simulink library "cmmi_lib"  (R2024a)
settings: Solver=VariableStepAuto  StartTime=0.0  StopTime=10.0  RelTol=1e-3
undefined symbols (not defined in the file): alloc_B, Keff, ss_x, ss_yaw, t200, t200_force_n, t200_pwm_n, Ts
libraries: ros2lib x12, MarineRoboticsLib x2, robotcorelib x1
settings Model: Creator=luka  LastModifiedBy=luka

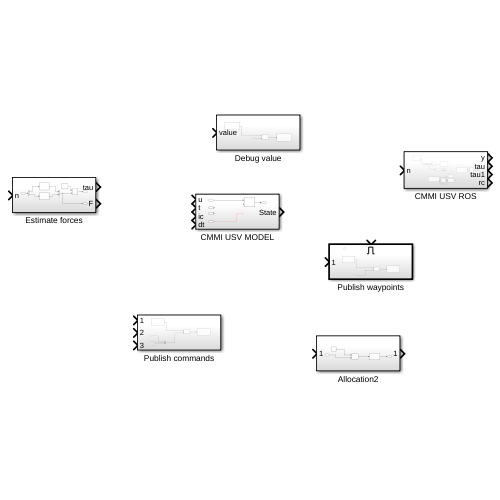
[thumbnail: Simulink's stored preview of the top-level diagram]
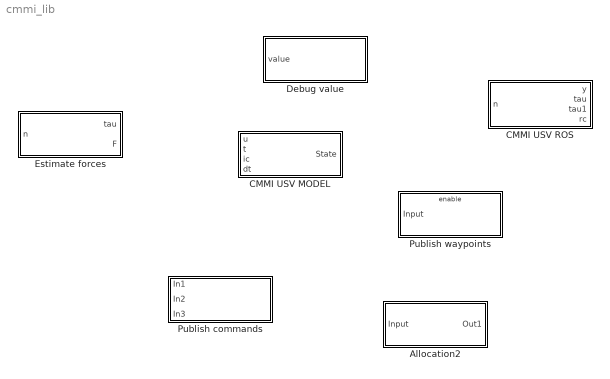
== system cmmi_lib ==
  Allocation2 : Subsystem
  CMMI USV MODEL : Subsystem
  CMMI USV ROS : Subsystem
  Debug value : Subsystem
  Estimate forces : Subsystem
  Publish commands : Subsystem
  Publish waypoints : Subsystem  TreatAsAtomicUnit=on

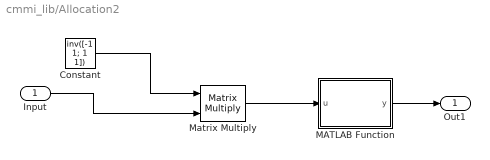
== system cmmi_lib/Allocation2 ==
  Input : Inport
  Constant : Constant  Value=inv([-1 1; 1 1])
  MATLAB Function : MATLAB Function  TreatAsAtomicUnit=on
  Matrix Multiply : Product  Multiplication=Matrix(*)
  Out1 : Outport
  wires:
  MATLAB Function/1(y) -> Out1/1
  Matrix Multiply/1 -> MATLAB Function/1(u)
  Input/1 -> Matrix Multiply/2
  Constant/1 -> Matrix Multiply/1

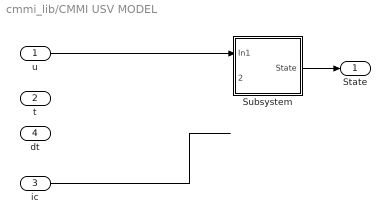
== system cmmi_lib/CMMI USV MODEL ==
  u : Inport
  t : Inport  Port=2
  ic : Inport  Port=3
  dt : Inport  Port=4
  Subsystem : Subsystem
  State : Outport
  wires:
  u/1 -> Subsystem/1(In1)
  Subsystem/1(State) -> State/1
  ic/1 -> ?

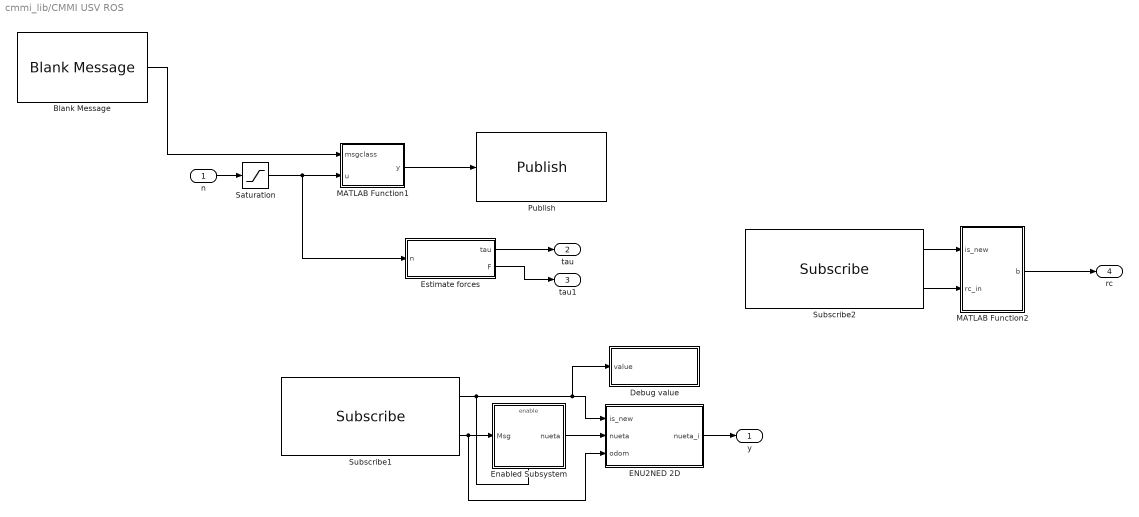
== system cmmi_lib/CMMI USV ROS ==
  n : Inport
  Blank Message : ros2lib/Blank Message  messageClass=Message  entityType=std_msgs/Float32MultiArray  messageType=std_msgs/Float32MultiArray  SampleTime=Ts
  Debug value : Subsystem  AncestorBlock=cmmi_lib/Debug value
  ENU2NED 2D : MATLAB Function  TreatAsAtomicUnit=on
  Enabled Subsystem : Subsystem  TreatAsAtomicUnit=on
  Estimate forces : Subsystem  AncestorBlock=cmmi_lib/Estimate forces
  MATLAB Function1 : MATLAB Function  TreatAsAtomicUnit=on
  MATLAB Function2 : MATLAB Function  TreatAsAtomicUnit=on  SystemSampleTime=Ts
  Publish : ros2lib/Publish  topicSource=Specify your own  topic=/pwm_in  messageType=std_msgs/Float32MultiArray  QOSHistory=Keep last  QOSDepth=1  QOSReliability=Reliable  QOSDurability=Volatile  QOSDeadline=Inf  QOSLifespan=Inf  QOSLiveliness=Automatic  QOSLeaseDuration=Inf  QOSAvoidROSNamespaceConventions=off
  Saturation : Saturate  UpperLimit=1  LowerLimit=-1
  Subscribe1 : ros2lib/Subscribe  topicSource=Specify your own  topic=/mavros/local_position/odom  messageType=nav_msgs/Odometry  sampleTime=0.05  QOSHistory=Keep last  QOSDepth=1  QOSReliability=Best effort  QOSDurability=Volatile  QOSDeadline=Inf  QOSLifespan=Inf  QOSLiveliness=Automatic  QOSLeaseDuration=Inf  QOSAvoidROSNamespaceConventions=off
  Subscribe2 : ros2lib/Subscribe  topicSource=Specify your own  topic=/rc_btns  messageType=std_msgs/Int8MultiArray  sampleTime=Ts  QOSHistory=Keep all  QOSDepth=1  QOSReliability=Best effort  QOSDurability=Volatile  QOSDeadline=Inf  QOSLifespan=Inf  QOSLiveliness=Automatic  QOSLeaseDuration=Inf  QOSAvoidROSNamespaceConventions=off
  y : Outport
  tau : Outport  Port=2
  tau1 : Outport  Port=3
  rc : Outport  Port=4
  wires:
  Saturation/1 -> MATLAB Function1/2(u), Estimate forces/1(n)
  ENU2NED 2D/1(nueta_i) -> y/1
  Enabled Subsystem/1(nueta) -> ENU2NED 2D/2(nueta)
  Subscribe1/1 -> Enabled Subsystem/Enable, ENU2NED 2D/1(is_new), Debug value/1(value)
  Subscribe1/2 -> Enabled Subsystem/1(Msg), ENU2NED 2D/3(odom)
  MATLAB Function2/1(b) -> rc/1
  Subscribe2/2 -> MATLAB Function2/2(rc_in)
  Subscribe2/1 -> MATLAB Function2/1(is_new)
  n/1 -> Saturation/1
  Blank Message/1 -> MATLAB Function1/1(msgclass)
  MATLAB Function1/1(y) -> Publish/1
  Estimate forces/1(tau) -> tau/1
  Estimate forces/2(F) -> tau1/1

== system cmmi_lib/Debug value ==
  value : Inport
  Blank Message : ros2lib/Blank Message  messageClass=Message  entityType=std_msgs/Float32MultiArray  messageType=std_msgs/Float32MultiArray  SampleTime=Ts
  MATLAB Function1 : MATLAB Function  TreatAsAtomicUnit=on
  Publish : ros2lib/Publish  topicSource=Specify your own  topic=debug  messageType=std_msgs/Float32MultiArray  QOSHistory=Keep last  QOSDepth=1  QOSReliability=Reliable  QOSDurability=Volatile  QOSDeadline=Inf  QOSLifespan=Inf  QOSLiveliness=Automatic  QOSLeaseDuration=Inf  QOSAvoidROSNamespaceConventions=off
  wires:
  value/1 -> MATLAB Function1/2(u)
  Blank Message/1 -> MATLAB Function1/1(msgclass)
  MATLAB Function1/1(y) -> Publish/1

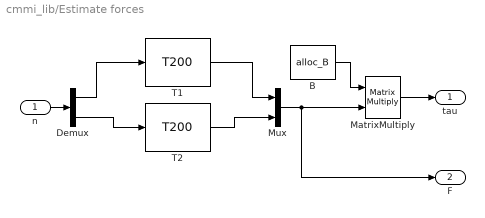
== system cmmi_lib/Estimate forces ==
  n : Inport
  B : Constant  Value=alloc_B
  Demux : Demux  Outputs=2
  MatrixMultiply : Product  Multiplication=Matrix(*)
  Mux : Mux  Inputs=2
  T1 : MarineRoboticsLib/T200  Keff=Keff(1)  Tm=Tm
  T2 : MarineRoboticsLib/T200  Keff=Keff(2)  Tm=Tm
  tau : Outport
  F : Outport  Port=2
  wires:
  MatrixMultiply/1 -> tau/1
  Demux/2 -> T2/1
  n/1 -> Demux/1
  Demux/1 -> T1/1
  Mux/1 -> MatrixMultiply/2, F/1
  T2/1 -> Mux/2
  B/1 -> MatrixMultiply/1
  T1/1 -> Mux/1

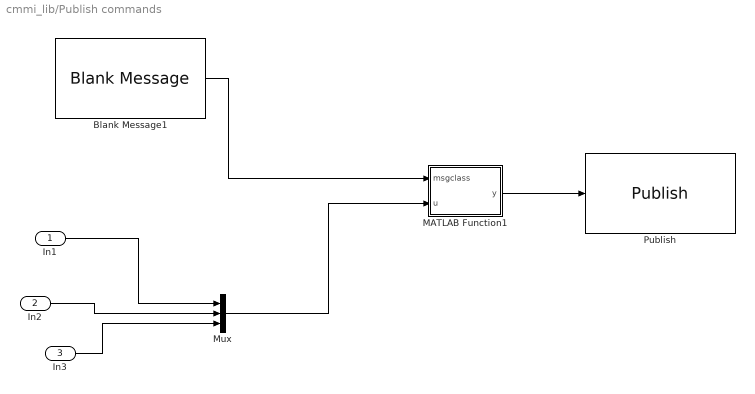
== system cmmi_lib/Publish commands ==
  In1 : Inport
  In2 : Inport  Port=2
  In3 : Inport  Port=3
  Blank Message1 : ros2lib/Blank Message  messageClass=Message  entityType=std_msgs/Float32MultiArray  messageType=std_msgs/Float32MultiArray  SampleTime=Ts
  MATLAB Function1 : MATLAB Function  TreatAsAtomicUnit=on
  Mux : Mux  Inputs=3
  Publish : ros2lib/Publish  topicSource=Specify your own  topic=/commands  messageType=std_msgs/Float32MultiArray  QOSHistory=Keep last  QOSDepth=1  QOSReliability=Reliable  QOSDurability=Volatile  QOSDeadline=Inf  QOSLifespan=Inf  QOSLiveliness=Automatic  QOSLeaseDuration=Inf  QOSAvoidROSNamespaceConventions=off
  wires:
  Blank Message1/1 -> MATLAB Function1/1(msgclass)
  MATLAB Function1/1(y) -> Publish/1
  Mux/1 -> MATLAB Function1/2(u)
  In1/1 -> Mux/1
  In2/1 -> Mux/2
  In3/1 -> Mux/3

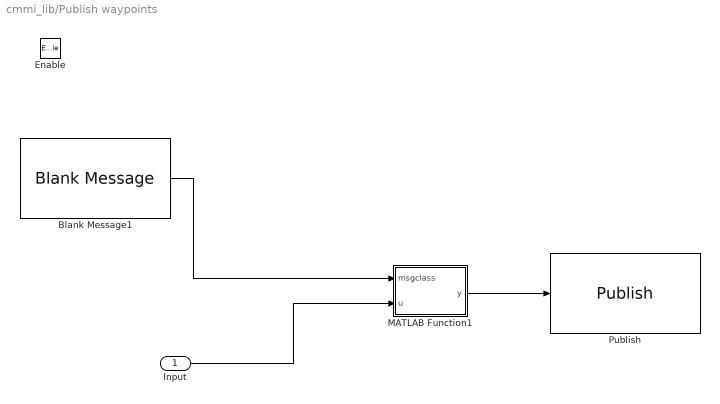
== system cmmi_lib/Publish waypoints ==
  Input : Inport
  Enable : EnablePort
  Blank Message1 : ros2lib/Blank Message  messageClass=Message  entityType=nav_msgs/Path  messageType=nav_msgs/Path  SampleTime=1
  MATLAB Function1 : MATLAB Function  TreatAsAtomicUnit=on
  Publish : ros2lib/Publish  topicSource=Specify your own  topic=/waypoints  messageType=nav_msgs/Path  QOSHistory=Keep last  QOSDepth=1  QOSReliability=Reliable  QOSDurability=Volatile  QOSDeadline=Inf  QOSLifespan=Inf  QOSLiveliness=Automatic  QOSLeaseDuration=Inf  QOSAvoidROSNamespaceConventions=off
  wires:
  Blank Message1/1 -> MATLAB Function1/1(msgclass)
  Input/1 -> MATLAB Function1/2(u)
  MATLAB Function1/1(y) -> Publish/1

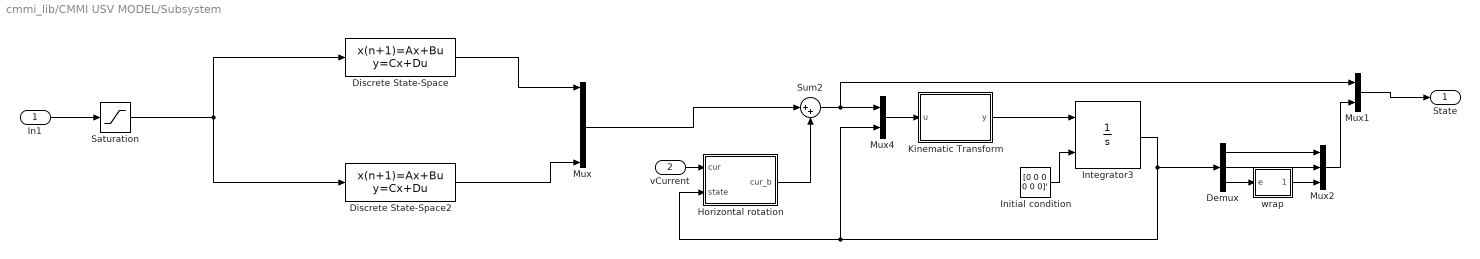
== system cmmi_lib/CMMI USV MODEL/Subsystem ==
  In1 : Inport
  vCurrent : Inport  Port=2
  Demux : Demux  Outputs=3
  Discrete State-Space : DiscreteStateSpace  A=ss_x.A  B=ss_x.B  C=ss_x.C  D=ss_x.D  SampleTime=ss_x.Ts
  Discrete State-Space2 : DiscreteStateSpace  A=ss_yaw.A  B=ss_yaw.B  C=ss_yaw.C  D=ss_yaw.D  SampleTime=ss_yaw.Ts
  Horizontal rotation : MATLAB Function  TreatAsAtomicUnit=on
  Initial condition : Constant  Value=[0 0 0 0 0 0]'
  Integrator3 : Integrator  InitialConditionSource=external
  Kinematic Transform : MATLAB Function  TreatAsAtomicUnit=on
  Mux : Mux  Inputs=6
  Mux1 : Mux  Inputs=2
  Mux2 : Mux  Inputs=3
  Mux4 : Mux  Inputs=2
  Saturation : Saturate  UpperLimit=1  LowerLimit=-1
  Sum2 : Sum  Inputs=|++
  wrap : MATLAB Function  TreatAsAtomicUnit=on
  State : Outport
  wires:
  In1/1 -> Saturation/1
  Discrete State-Space2/1 -> Mux/6
  Kinematic Transform/1(y) -> Integrator3/1
  Initial condition/1 -> Integrator3/2
  Sum2/1 -> Mux1/1, Mux4/1
  vCurrent/1 -> Horizontal rotation/1(cur)
  Mux4/1 -> Kinematic Transform/1(u)
  Integrator3/1 -> Demux/1, Horizontal rotation/2(state), Mux4/2
  Mux/1 -> Sum2/1
  Horizontal rotation/1(cur_b) -> Sum2/2
  Mux1/1 -> State/1
  Discrete State-Space/1 -> Mux/1
  Demux/3 -> wrap/1(e)
  wrap/1(ew) -> Mux2/3
  Demux/1 -> Mux2/1
  Demux/2 -> Mux2/2
  Mux2/1 -> Mux1/2
  Saturation/1 -> Discrete State-Space2/1, Discrete State-Space/1

== system cmmi_lib/CMMI USV ROS/Debug value ==
  value : Inport
  Blank Message : ros2lib/Blank Message  messageClass=Message  entityType=std_msgs/Float32MultiArray  messageType=std_msgs/Float32MultiArray  SampleTime=Ts
  MATLAB Function1 : MATLAB Function  TreatAsAtomicUnit=on
  Publish : ros2lib/Publish  topicSource=Specify your own  topic=debug_isnew  messageType=std_msgs/Float32MultiArray  QOSHistory=Keep last  QOSDepth=1  QOSReliability=Reliable  QOSDurability=Volatile  QOSDeadline=Inf  QOSLifespan=Inf  QOSLiveliness=Automatic  QOSLeaseDuration=Inf  QOSAvoidROSNamespaceConventions=off
  wires:
  MATLAB Function1/1(y) -> Publish/1
  Blank Message/1 -> MATLAB Function1/1(msgclass)
  value/1 -> MATLAB Function1/2(u)

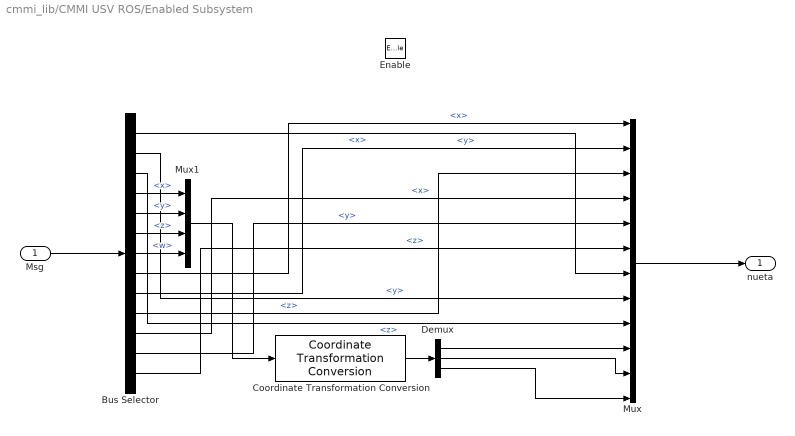
== system cmmi_lib/CMMI USV ROS/Enabled Subsystem ==
  Msg : Inport
  Enable : EnablePort
  Bus Selector : BusSelector  OutputSignals=pose.pose.position.x,pose.pose.position.y,pose.pose.position.z,pose.pose.orientation.x,pose.pose.orientation.y,pose.pose.orientation.z,pose.pose.orientation.w,twist.twist.linear.x,twist.twist.linear.y,twist.twist.linear.z,twist.twist.angular.x,twist.twist.angular.y,twist.twist.angular.z
  Coordinate Transformation Conversion : robotcorelib/Coordinate Transformation Conversion  InputRepresentation=Quaternion  InputEulerSequence=ZYX  ShowTrVecInputPort=on  OutputRepresentation=Euler Angles  OutputEulerSequence=ZYX  ShowTrVecOutputPort=on  SimulateUsing=Code generation
      settings: LibrarySourceBlock=roslib/Utilities/Coordinate Transformation Conversion
  Demux : Demux  Outputs=3
  Mux : Mux  Inputs=12
  Mux1 : Mux
  nueta : Outport
  wires:
  Bus Selector/12 -> Mux/5  "<y>"
  Bus Selector/11 -> Mux/4  "<x>"
  Bus Selector/10 -> Mux/3  "<z>"
  Demux/1 -> Mux/10
  Demux/2 -> Mux/11
  Bus Selector/3 -> Mux/9  "<z>"
  Msg/1 -> Bus Selector/1
  Bus Selector/4 -> Mux1/1  "<x>"
  Bus Selector/5 -> Mux1/2  "<y>"
  Bus Selector/6 -> Mux1/3  "<z>"
  Bus Selector/7 -> Mux1/4  "<w>"
  Mux1/1 -> Coordinate Transformation Conversion/1
  Bus Selector/2 -> Mux/8  "<y>"
  Bus Selector/1 -> Mux/7  "<x>"
  Coordinate Transformation Conversion/1 -> Demux/1
  Bus Selector/8 -> Mux/1  "<x>"
  Bus Selector/9 -> Mux/2  "<y>"
  Bus Selector/13 -> Mux/6  "<z>"
  Mux/1 -> nueta/1
  Demux/3 -> Mux/12

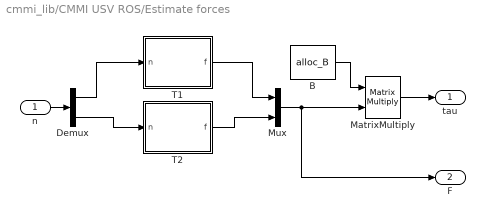
== system cmmi_lib/CMMI USV ROS/Estimate forces ==
  n : Inport
  B : Constant  Value=alloc_B
  Demux : Demux  Outputs=2
  MatrixMultiply : Product  Multiplication=Matrix(*)
  Mux : Mux  Inputs=2
  T1 : Subsystem  mask(T200){Keff=t200(1).Keff, Tm=t200(1).Tm}
      mask prompts: Keff "Efficiency"; Tm "ESC time constant (Tm)"
      mask help: This simulink block simulates a Blue Robotics T200 thruster on 14V controlled input. The efficiancy parameter given from [0,1] additionally decreases the force output of the thruster. The ESC reaction time is the time constant of the PT1 element included in the model. Put the time constant to zero to have instantaneous response.
      mask Display: image('$imagefile'); % Use "Edit Image" on toolstrip to change.
  T2 : Subsystem  mask(T200){Keff=t200(2).Keff, Tm=t200(2).Tm}
      mask prompts: Keff "Efficiency"; Tm "ESC time constant (Tm)"
      mask help: This simulink block simulates a Blue Robotics T200 thruster on 14V controlled input. The efficiancy parameter given from [0,1] additionally decreases the force output of the thruster. The ESC reaction time is the time constant of the PT1 element included in the model. Put the time constant to zero to have instantaneous response.
      mask Display: image('$imagefile'); % Use "Edit Image" on toolstrip to change.
  tau : Outport
  F : Outport  Port=2
  wires:
  T1/1(f) -> Mux/1
  B/1 -> MatrixMultiply/1
  T2/1(f) -> Mux/2
  Mux/1 -> F/1, MatrixMultiply/2
  Demux/1 -> T1/1(n)
  n/1 -> Demux/1
  Demux/2 -> T2/1(n)
  MatrixMultiply/1 -> tau/1

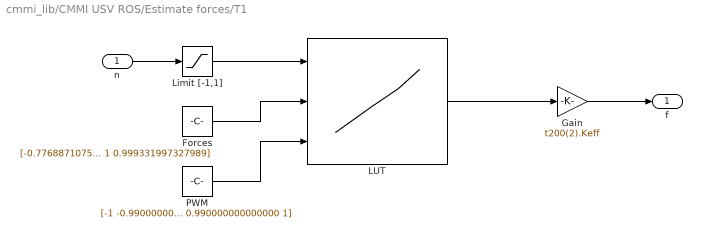
== system cmmi_lib/CMMI USV ROS/Estimate forces/T1 ==
  n : Inport
  Forces : Constant  Value=|
      | [-0.776887107548430
      | -0.772545090180361
      | -0.771543086172345
      | -0.762525050100200
      | -0.751503006012024
      | -0.741482965931864
      | -0.727454909819639
      | -0.717434869739479
      | -0.704408817635270
      | -0.693386773547094
      | -0.684368737474950
      | -0.675350701402806
      | -0.663326653306613
      | -0.649298597194389
      | -0.637274549098196
      | -0.629258517034068
      | -0.614228456913828
      | -0.610220440881764
      | -0.594188376753507
      | -0.584168336673347
      | -0.573146292585170
      | -0.558116232464930
      | -0.550100200400802
      | -0.542084168336673
      | -0.532064128256513
      | -0.519038076152305
      | -0.516032064128256
      | -0.498997995991984
      | -0.486973947895792
      | -0.480961923847695
      | -0.467935871743487
      | -0.453907815631262
      | -0.447895791583166
      | -0.438877755511022
      | -0.421843687374750
      | -0.417835671342685
      | -0.401803607214429
      | -0.389779559118237
      | -0.379759519038076
      | -0.371743486973948
      | -0.360721442885772
      | -0.348697394789579
      | -0.345691382765531
      | -0.335671342685371
      | -0.326653306613226
      | -0.318637274549098
      | -0.309619238476954
      | -0.302605210420842
      | -0.292585170340681
      | -0.283567134268537
      | -0.273547094188377
      | -0.263527054108217
      | -0.257515030060120
      | -0.248496993987976
      | -0.240480961923848
      | -0.232464929859719
      | -0.224448897795591
      | -0.217434869739479
      | -0.210420841683367
      | -0.202404809619238
      | -0.195390781563126
      | -0.187374749498998
      | -0.178356713426854
      | -0.169338677354709
      | -0.163326653306613
      | -0.155310621242485
      | -0.150300601202405
      | -0.143286573146293
      | -0.137274549098196
      | -0.129258517034068
      | -0.121242484969940
      | -0.114228456913828
      | -0.108216432865731
      | -0.102204408817635
      | -0.0941883767535070
      | -0.0881763527054108
      | -0.0821643286573146
      | -0.0771543086172345
      | -0.0701402805611222
      | -0.0631262525050100
      | -0.0571142284569138
      | -0.0521042084168337
      | -0.0460921843687375
      | -0.0410821643286573
      | -0.0360721442885772
      | -0.0320641282565130
      | -0.0270541082164329
      | -0.0220440881763527
      | -0.0180360721442886
      | -0.0150300601202405
      | -0.0100200400801603
      | -0.00701402805611223
      | 0
      | 0
      | 0
      | 0
      | 0
      | 0
      | 0
      | 0
      | 0
      | 0
      | 0
      | 0
      | 0
      | 0
      | 0
      | 0
      | 0
      | 0.0100200400801603
      | 0.0140280561122245
      | 0.0180360721442886
      | 0.0220440881763527
      | 0.0270541082164329
      | 0.0320641282565130
      | 0.0390781563126253
      | 0.0440881763527054
      | 0.0501002004008016
      | 0.0581162324649299
      | 0.0641282565130261
      | 0.0721442885771543
      | 0.0801603206412826
      | 0.0871743486973948
      | 0.0941883767535070
      | 0.102204408817635
      | 0.110220440881764
      | 0.117234468937876
      | 0.127254509018036
      | 0.137274549098196
      | 0.142284569138277
      | 0.152304609218437
      | 0.160320641282565
      | 0.169338677354709
      | 0.182364729458918
      | 0.187374749498998
      | 0.196392785571142
      | 0.203406813627254
      | 0.213426853707415
      | 0.220440881763527
      | 0.232464929859719
      | 0.241482965931864
      | 0.252505010020040
      | 0.265531062124249
      | 0.272545090180361
      | 0.282565130260521
      | 0.292585170340681
      | 0.301603206412826
      | 0.310621242484970
      | 0.322645290581162
      | 0.333667334669339
      | 0.342685370741483
      | 0.354709418837675
      | 0.364729458917836
      | 0.377755511022044
      | 0.388777555110220
      | 0.400801603206413
      | 0.408817635270541
      | 0.421843687374750
      | 0.433867735470942
      | 0.442885771543086
      | 0.460921843687375
      | 0.467935871743487
      | 0.476953907815631
      | 0.495991983967936
      | 0.501002004008016
      | 0.517034068136273
      | 0.536072144288577
      | 0.553106212424850
      | 0.566132264529058
      | 0.582164328657315
      | 0.587174348697395
      | 0.609218436873748
      | 0.614228456913828
      | 0.636272545090180
      | 0.648296593186373
      | 0.661322645290581
      | 0.673346693386774
      | 0.691382765531062
      | 0.704408817635271
      | 0.714428857715431
      | 0.734468937875751
      | 0.742484969939880
      | 0.755511022044088
      | 0.771543086172345
      | 0.787575150300601
      | 0.800601202404810
      | 0.814629258517034
      | 0.832665330661323
      | 0.847695390781563
      | 0.866733466933868
      | 0.879759519038076
      | 0.889779559118237
      | 0.907815631262525
      | 0.917835671342685
      | 0.930861723446894
      | 0.950901803607214
      | 0.967935871743487
      | 0.976953907815631
      | 0.995991983967936
      | 1
      | 0.999331997327989]
  Gain : Gain  Gain=t200(2).Keff
  LUT : Lookup_n-D  NumberOfTableDimensions=1  BreakpointsForDimension1Source=Input port  BreakpointsForDimension1=t200_pwm_n  TableSource=Input port  Table=t200_force_n  InternalRulePriority=Speed  RndMeth=Simplest
      settings: InputPortMap=u0,p221,p5
  Limit [-1,1] : Saturate  UpperLimit=1  LowerLimit=-1
  PWM : Constant  Value=|
      | [-1
      | -0.990000000000000
      | -0.980000000000000
      | -0.970000000000000
      | -0.960000000000000
      | -0.950000000000000
      | -0.940000000000000
      | -0.930000000000000
      | -0.920000000000000
      | -0.910000000000000
      | -0.900000000000000
      | -0.890000000000000
      | -0.880000000000000
      | -0.870000000000000
      | -0.860000000000000
      | -0.850000000000000
      | -0.840000000000000
      | -0.830000000000000
      | -0.820000000000000
      | -0.810000000000000
      | -0.800000000000000
      | -0.790000000000000
      | -0.780000000000000
      | -0.770000000000000
      | -0.760000000000000
      | -0.750000000000000
      | -0.740000000000000
      | -0.730000000000000
      | -0.720000000000000
      | -0.710000000000000
      | -0.700000000000000
      | -0.690000000000000
      | -0.680000000000000
      | -0.670000000000000
      | -0.660000000000000
      | -0.650000000000000
      | -0.640000000000000
      | -0.630000000000000
      | -0.620000000000000
      | -0.610000000000000
      | -0.600000000000000
      | -0.590000000000000
      | -0.580000000000000
      | -0.570000000000000
      | -0.560000000000000
      | -0.550000000000000
      | -0.540000000000000
      | -0.530000000000000
      | -0.520000000000000
      | -0.510000000000000
      | -0.500000000000000
      | -0.490000000000000
      | -0.480000000000000
      | -0.470000000000000
      | -0.460000000000000
      | -0.450000000000000
      | -0.440000000000000
      | -0.430000000000000
      | -0.420000000000000
      | -0.410000000000000
      | -0.400000000000000
      | -0.390000000000000
      | -0.380000000000000
      | -0.370000000000000
      | -0.360000000000000
      | -0.350000000000000
      | -0.340000000000000
      | -0.330000000000000
      | -0.320000000000000
      | -0.310000000000000
      | -0.300000000000000
      | -0.290000000000000
      | -0.280000000000000
      | -0.270000000000000
      | -0.260000000000000
      | -0.250000000000000
      | -0.240000000000000
      | -0.230000000000000
      | -0.220000000000000
      | -0.210000000000000
      | -0.200000000000000
      | -0.190000000000000
      | -0.180000000000000
      | -0.170000000000000
      | -0.160000000000000
      | -0.150000000000000
      | -0.140000000000000
      | -0.130000000000000
      | -0.120000000000000
      | -0.110000000000000
      | -0.100000000000000
      | -0.0900000000000000
      | -0.0800000000000000
      | -0.0700000000000000
      | -0.0600000000000000
      | -0.0500000000000000
      | -0.0400000000000000
      | -0.0300000000000000
      | -0.0200000000000000
      | -0.0100000000000000
      | 0
      | 0.0100000000000000
      | 0.0200000000000000
      | 0.0300000000000000
      | 0.0400000000000000
      | 0.0500000000000000
      | 0.0600000000000000
      | 0.0700000000000000
      | 0.0800000000000000
      | 0.0900000000000000
      | 0.100000000000000
      | 0.110000000000000
      | 0.120000000000000
      | 0.130000000000000
      | 0.140000000000000
      | 0.150000000000000
      | 0.160000000000000
      | 0.170000000000000
      | 0.180000000000000
      | 0.190000000000000
      | 0.200000000000000
      | 0.210000000000000
      | 0.220000000000000
      | 0.230000000000000
      | 0.240000000000000
      | 0.250000000000000
      | 0.260000000000000
      | 0.270000000000000
      | 0.280000000000000
      | 0.290000000000000
      | 0.300000000000000
      | 0.310000000000000
      | 0.320000000000000
      | 0.330000000000000
      | 0.340000000000000
      | 0.350000000000000
      | 0.360000000000000
      | 0.370000000000000
      | 0.380000000000000
      | 0.390000000000000
      | 0.400000000000000
      | 0.410000000000000
      | 0.420000000000000
      | 0.430000000000000
      | 0.440000000000000
      | 0.450000000000000
      | 0.460000000000000
      | 0.470000000000000
      | 0.480000000000000
      | 0.490000000000000
      | 0.500000000000000
      | 0.510000000000000
      | 0.520000000000000
      | 0.530000000000000
      | 0.540000000000000
      | 0.550000000000000
      | 0.560000000000000
      | 0.570000000000000
      | 0.580000000000000
      | 0.590000000000000
      | 0.600000000000000
      | 0.610000000000000
      | 0.620000000000000
      | 0.630000000000000
      | 0.640000000000000
      | 0.650000000000000
      | 0.660000000000000
      | 0.670000000000000
      | 0.680000000000000
      | 0.690000000000000
      | 0.700000000000000
      | 0.710000000000000
      | 0.720000000000000
      | 0.730000000000000
      | 0.740000000000000
      | 0.750000000000000
      | 0.760000000000000
      | 0.770000000000000
      | 0.780000000000000
      | 0.790000000000000
      | 0.800000000000000
      | 0.810000000000000
      | 0.820000000000000
      | 0.830000000000000
      | 0.840000000000000
      | 0.850000000000000
      | 0.860000000000000
      | 0.870000000000000
      | 0.880000000000000
      | 0.890000000000000
      | 0.900000000000000
      | 0.910000000000000
      | 0.920000000000000
      | 0.930000000000000
      | 0.940000000000000
      | 0.950000000000000
      | 0.960000000000000
      | 0.970000000000000
      | 0.980000000000000
      | 0.990000000000000
      | 1]
  f : Outport
  wires:
  PWM/1 -> LUT/3
  Forces/1 -> LUT/2
  Gain/1 -> f/1
  n/1 -> Limit [-1,1]/1
  LUT/1 -> Gain/1
  Limit [-1,1]/1 -> LUT/1

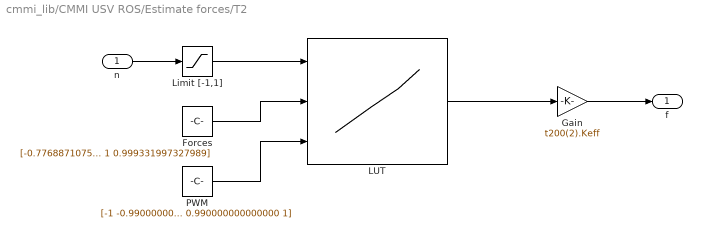
== system cmmi_lib/CMMI USV ROS/Estimate forces/T2 ==
  n : Inport
  Forces : Constant  Value=|
      | [-0.776887107548430
      | -0.772545090180361
      | -0.771543086172345
      | -0.762525050100200
      | -0.751503006012024
      | -0.741482965931864
      | -0.727454909819639
      | -0.717434869739479
      | -0.704408817635270
      | -0.693386773547094
      | -0.684368737474950
      | -0.675350701402806
      | -0.663326653306613
      | -0.649298597194389
      | -0.637274549098196
      | -0.629258517034068
      | -0.614228456913828
      | -0.610220440881764
      | -0.594188376753507
      | -0.584168336673347
      | -0.573146292585170
      | -0.558116232464930
      | -0.550100200400802
      | -0.542084168336673
      | -0.532064128256513
      | -0.519038076152305
      | -0.516032064128256
      | -0.498997995991984
      | -0.486973947895792
      | -0.480961923847695
      | -0.467935871743487
      | -0.453907815631262
      | -0.447895791583166
      | -0.438877755511022
      | -0.421843687374750
      | -0.417835671342685
      | -0.401803607214429
      | -0.389779559118237
      | -0.379759519038076
      | -0.371743486973948
      | -0.360721442885772
      | -0.348697394789579
      | -0.345691382765531
      | -0.335671342685371
      | -0.326653306613226
      | -0.318637274549098
      | -0.309619238476954
      | -0.302605210420842
      | -0.292585170340681
      | -0.283567134268537
      | -0.273547094188377
      | -0.263527054108217
      | -0.257515030060120
      | -0.248496993987976
      | -0.240480961923848
      | -0.232464929859719
      | -0.224448897795591
      | -0.217434869739479
      | -0.210420841683367
      | -0.202404809619238
      | -0.195390781563126
      | -0.187374749498998
      | -0.178356713426854
      | -0.169338677354709
      | -0.163326653306613
      | -0.155310621242485
      | -0.150300601202405
      | -0.143286573146293
      | -0.137274549098196
      | -0.129258517034068
      | -0.121242484969940
      | -0.114228456913828
      | -0.108216432865731
      | -0.102204408817635
      | -0.0941883767535070
      | -0.0881763527054108
      | -0.0821643286573146
      | -0.0771543086172345
      | -0.0701402805611222
      | -0.0631262525050100
      | -0.0571142284569138
      | -0.0521042084168337
      | -0.0460921843687375
      | -0.0410821643286573
      | -0.0360721442885772
      | -0.0320641282565130
      | -0.0270541082164329
      | -0.0220440881763527
      | -0.0180360721442886
      | -0.0150300601202405
      | -0.0100200400801603
      | -0.00701402805611223
      | 0
      | 0
      | 0
      | 0
      | 0
      | 0
      | 0
      | 0
      | 0
      | 0
      | 0
      | 0
      | 0
      | 0
      | 0
      | 0
      | 0
      | 0.0100200400801603
      | 0.0140280561122245
      | 0.0180360721442886
      | 0.0220440881763527
      | 0.0270541082164329
      | 0.0320641282565130
      | 0.0390781563126253
      | 0.0440881763527054
      | 0.0501002004008016
      | 0.0581162324649299
      | 0.0641282565130261
      | 0.0721442885771543
      | 0.0801603206412826
      | 0.0871743486973948
      | 0.0941883767535070
      | 0.102204408817635
      | 0.110220440881764
      | 0.117234468937876
      | 0.127254509018036
      | 0.137274549098196
      | 0.142284569138277
      | 0.152304609218437
      | 0.160320641282565
      | 0.169338677354709
      | 0.182364729458918
      | 0.187374749498998
      | 0.196392785571142
      | 0.203406813627254
      | 0.213426853707415
      | 0.220440881763527
      | 0.232464929859719
      | 0.241482965931864
      | 0.252505010020040
      | 0.265531062124249
      | 0.272545090180361
      | 0.282565130260521
      | 0.292585170340681
      | 0.301603206412826
      | 0.310621242484970
      | 0.322645290581162
      | 0.333667334669339
      | 0.342685370741483
      | 0.354709418837675
      | 0.364729458917836
      | 0.377755511022044
      | 0.388777555110220
      | 0.400801603206413
      | 0.408817635270541
      | 0.421843687374750
      | 0.433867735470942
      | 0.442885771543086
      | 0.460921843687375
      | 0.467935871743487
      | 0.476953907815631
      | 0.495991983967936
      | 0.501002004008016
      | 0.517034068136273
      | 0.536072144288577
      | 0.553106212424850
      | 0.566132264529058
      | 0.582164328657315
      | 0.587174348697395
      | 0.609218436873748
      | 0.614228456913828
      | 0.636272545090180
      | 0.648296593186373
      | 0.661322645290581
      | 0.673346693386774
      | 0.691382765531062
      | 0.704408817635271
      | 0.714428857715431
      | 0.734468937875751
      | 0.742484969939880
      | 0.755511022044088
      | 0.771543086172345
      | 0.787575150300601
      | 0.800601202404810
      | 0.814629258517034
      | 0.832665330661323
      | 0.847695390781563
      | 0.866733466933868
      | 0.879759519038076
      | 0.889779559118237
      | 0.907815631262525
      | 0.917835671342685
      | 0.930861723446894
      | 0.950901803607214
      | 0.967935871743487
      | 0.976953907815631
      | 0.995991983967936
      | 1
      | 0.999331997327989]
  Gain : Gain  Gain=t200(2).Keff
  LUT : Lookup_n-D  NumberOfTableDimensions=1  BreakpointsForDimension1Source=Input port  BreakpointsForDimension1=t200_pwm_n  TableSource=Input port  Table=t200_force_n  InternalRulePriority=Speed  RndMeth=Simplest
      settings: InputPortMap=u0,p221,p5
  Limit [-1,1] : Saturate  UpperLimit=1  LowerLimit=-1
  PWM : Constant  Value=|
      | [-1
      | -0.990000000000000
      | -0.980000000000000
      | -0.970000000000000
      | -0.960000000000000
      | -0.950000000000000
      | -0.940000000000000
      | -0.930000000000000
      | -0.920000000000000
      | -0.910000000000000
      | -0.900000000000000
      | -0.890000000000000
      | -0.880000000000000
      | -0.870000000000000
      | -0.860000000000000
      | -0.850000000000000
      | -0.840000000000000
      | -0.830000000000000
      | -0.820000000000000
      | -0.810000000000000
      | -0.800000000000000
      | -0.790000000000000
      | -0.780000000000000
      | -0.770000000000000
      | -0.760000000000000
      | -0.750000000000000
      | -0.740000000000000
      | -0.730000000000000
      | -0.720000000000000
      | -0.710000000000000
      | -0.700000000000000
      | -0.690000000000000
      | -0.680000000000000
      | -0.670000000000000
      | -0.660000000000000
      | -0.650000000000000
      | -0.640000000000000
      | -0.630000000000000
      | -0.620000000000000
      | -0.610000000000000
      | -0.600000000000000
      | -0.590000000000000
      | -0.580000000000000
      | -0.570000000000000
      | -0.560000000000000
      | -0.550000000000000
      | -0.540000000000000
      | -0.530000000000000
      | -0.520000000000000
      | -0.510000000000000
      | -0.500000000000000
      | -0.490000000000000
      | -0.480000000000000
      | -0.470000000000000
      | -0.460000000000000
      | -0.450000000000000
      | -0.440000000000000
      | -0.430000000000000
      | -0.420000000000000
      | -0.410000000000000
      | -0.400000000000000
      | -0.390000000000000
      | -0.380000000000000
      | -0.370000000000000
      | -0.360000000000000
      | -0.350000000000000
      | -0.340000000000000
      | -0.330000000000000
      | -0.320000000000000
      | -0.310000000000000
      | -0.300000000000000
      | -0.290000000000000
      | -0.280000000000000
      | -0.270000000000000
      | -0.260000000000000
      | -0.250000000000000
      | -0.240000000000000
      | -0.230000000000000
      | -0.220000000000000
      | -0.210000000000000
      | -0.200000000000000
      | -0.190000000000000
      | -0.180000000000000
      | -0.170000000000000
      | -0.160000000000000
      | -0.150000000000000
      | -0.140000000000000
      | -0.130000000000000
      | -0.120000000000000
      | -0.110000000000000
      | -0.100000000000000
      | -0.0900000000000000
      | -0.0800000000000000
      | -0.0700000000000000
      | -0.0600000000000000
      | -0.0500000000000000
      | -0.0400000000000000
      | -0.0300000000000000
      | -0.0200000000000000
      | -0.0100000000000000
      | 0
      | 0.0100000000000000
      | 0.0200000000000000
      | 0.0300000000000000
      | 0.0400000000000000
      | 0.0500000000000000
      | 0.0600000000000000
      | 0.0700000000000000
      | 0.0800000000000000
      | 0.0900000000000000
      | 0.100000000000000
      | 0.110000000000000
      | 0.120000000000000
      | 0.130000000000000
      | 0.140000000000000
      | 0.150000000000000
      | 0.160000000000000
      | 0.170000000000000
      | 0.180000000000000
      | 0.190000000000000
      | 0.200000000000000
      | 0.210000000000000
      | 0.220000000000000
      | 0.230000000000000
      | 0.240000000000000
      | 0.250000000000000
      | 0.260000000000000
      | 0.270000000000000
      | 0.280000000000000
      | 0.290000000000000
      | 0.300000000000000
      | 0.310000000000000
      | 0.320000000000000
      | 0.330000000000000
      | 0.340000000000000
      | 0.350000000000000
      | 0.360000000000000
      | 0.370000000000000
      | 0.380000000000000
      | 0.390000000000000
      | 0.400000000000000
      | 0.410000000000000
      | 0.420000000000000
      | 0.430000000000000
      | 0.440000000000000
      | 0.450000000000000
      | 0.460000000000000
      | 0.470000000000000
      | 0.480000000000000
      | 0.490000000000000
      | 0.500000000000000
      | 0.510000000000000
      | 0.520000000000000
      | 0.530000000000000
      | 0.540000000000000
      | 0.550000000000000
      | 0.560000000000000
      | 0.570000000000000
      | 0.580000000000000
      | 0.590000000000000
      | 0.600000000000000
      | 0.610000000000000
      | 0.620000000000000
      | 0.630000000000000
      | 0.640000000000000
      | 0.650000000000000
      | 0.660000000000000
      | 0.670000000000000
      | 0.680000000000000
      | 0.690000000000000
      | 0.700000000000000
      | 0.710000000000000
      | 0.720000000000000
      | 0.730000000000000
      | 0.740000000000000
      | 0.750000000000000
      | 0.760000000000000
      | 0.770000000000000
      | 0.780000000000000
      | 0.790000000000000
      | 0.800000000000000
      | 0.810000000000000
      | 0.820000000000000
      | 0.830000000000000
      | 0.840000000000000
      | 0.850000000000000
      | 0.860000000000000
      | 0.870000000000000
      | 0.880000000000000
      | 0.890000000000000
      | 0.900000000000000
      | 0.910000000000000
      | 0.920000000000000
      | 0.930000000000000
      | 0.940000000000000
      | 0.950000000000000
      | 0.960000000000000
      | 0.970000000000000
      | 0.980000000000000
      | 0.990000000000000
      | 1]
  f : Outport
  wires:
  PWM/1 -> LUT/3
  Forces/1 -> LUT/2
  Gain/1 -> f/1
  n/1 -> Limit [-1,1]/1
  LUT/1 -> Gain/1
  Limit [-1,1]/1 -> LUT/1

== matlab function cmmi_lib/CMMI USV MODEL/Subsystem/Horizontal rotation ==
  data: cur input; cur_b output; state input
function cur_b = fcn(cur, state)
cur_b = zeros(6,1);
Psi = state(6,1);
R_z_psi = [cos(Psi) sin(Psi); -sin(Psi) cos(Psi)];

cur_ne_b = R_z_psi*cur;
cur_b(1) = cur_ne_b(1);
cur_b(2) = cur_ne_b(2);

== matlab function cmmi_lib/Publish commands/MATLAB Function1 ==
  data: msgclass input; u input; y output Bus: SL_Bus_std_msgs_Float32MultiArray
function y = fcn(msgclass, u)

% blank message input
msg = msgclass();

% assign pwm values into data field
msg.data(1:numel(u)) = reshape(u,[],1);

% all other fields must be assigned to complete the message
msg.data_SL_Info.CurrentLength = uint32(numel(u));
msg.layout.dim(1).size = uint32(size(u,1));

y = msg;

== matlab function cmmi_lib/CMMI USV ROS/Debug value/MATLAB Function1 ==
  data: msgclass input; u input; y output Bus: SL_Bus_std_msgs_Float32MultiArray
function y = fcn(msgclass, u)

% blank message input
msg = msgclass();


% all other fields must be assigned to complete the message
msg.data_SL_Info.CurrentLength = uint32(numel(u));
msg.layout.dim_SL_Info.CurrentLength = uint32(1);
msg.layout.dim(1).size = uint32(size(u,1));

% assign pwm values into data field
msg.data(1:numel(u)) = reshape(u,[],1);


y = msg;

== matlab function cmmi_lib/CMMI USV ROS/MATLAB Function1 ==
  data: msgclass input; u input; y output Bus: SL_Bus_std_msgs_Float32MultiArray
function y = fcn(msgclass, u)

% blank message input
msg = msgclass();


% all other fields must be assigned to complete the message
msg.data_SL_Info.CurrentLength = uint32(numel(u));
msg.layout.dim_SL_Info.CurrentLength = uint32(1);
msg.layout.dim(1).size = uint32(size(u,1));

% assign pwm values into data field
msg.data(1:numel(u)) = reshape(u,[],1);


y = msg;

== matlab function cmmi_lib/CMMI USV ROS/ENU2NED 2D ==
  data: is_new input; nueta_i output; nueta input; odom input
function nueta_i = enu2ned2d(is_new, nueta, odom)
% % Just do coordinate swap
% psi_ned = pi/2-psi_enu;
% 
% psi_ned = mod(psi_ned, 2*pi);
% 
% if psi_ned > pi
%    psi_ned = -2*pi + psi_ned;
% elseif psi_ned <= -pi 
%    psi_ned = 2*pi + psi_ned;
% end
% 
% 
% eta = [y_enu; x_enu; psi_ned];
% nu = [u_enu; -v_enu; -r_enu;];

persistent f_t s_t f s t start_t

    nueta_i = [0,0,0,0,0,0,0,0,0,0,0,0]';

    if isempty(f_t)
        f_t = -1;
        s_t = -1;
        f = nueta;
        s = nueta;
        start_t = 0;
        t = 0;
    end

    if is_new
        s_t = f_t;
        s = f;
        f_t = double(odom.header.stamp.sec) + 1e-9 * double(odom.header.stamp.nanosec);
        f = nueta;
        if start_t == 0
            start_t = f_t;
        end
    end
    t = t + 0.05;

    if isempty(f_t)
        return
    end
    
    if s_t == -1
        nueta_i = f;
        return
    end
    
    dt = (s_t - f_t);
    if dt > 0.001
        k = (s - f) / (s_t - f_t);
        dt = max(t - (f_t - start_t), 0);
        nueta_i = f + k*dt;
    else
        nueta_i = f;
    end

== matlab function cmmi_lib/Debug value/MATLAB Function1 ==
  data: msgclass input; u input; y output Bus: SL_Bus_std_msgs_Float32MultiArray
function y = fcn(msgclass, u)

% blank message input
msg = msgclass();


% all other fields must be assigned to complete the message
msg.data_SL_Info.CurrentLength = uint32(numel(u));
msg.layout.dim_SL_Info.CurrentLength = uint32(1);
msg.layout.dim(1).size = uint32(size(u,1));

% assign pwm values into data field
msg.data(1:numel(u)) = reshape(u,[],1);


y = msg;

== matlab function cmmi_lib/Publish waypoints/MATLAB Function1 ==
  data: msgclass input; u input; y output Bus: SL_Bus_nav_msgs_Path
function y = fcn(msgclass, u)

% blank message input
msg = msgclass();

num_points = 5;
% num_points = 127;
msg.poses_SL_Info.CurrentLength = uint32(num_points);
for i=1:num_points
    msg.poses(i).pose.position.x = u(i, 1);
    msg.poses(i).pose.position.y = u(i, 2);
    msg.poses(i).pose.orientation.z = u(i, 3);
end
y = msg;

== matlab function cmmi_lib/CMMI USV MODEL/Subsystem/Kinematic Transform ==
  data: u input; y output
function y = fcn(u)
%#codegen
if (length(u)<12) 
    y = zeros(12,1);
    return;
end

input = u;
% Read inputs
u = input(1,1);
v = input(2,1);
w = input(3,1);
p = input(4,1);
q = input(5,1);
r = input(6,1);

%x = input(7,1);
%y = input(8,1);
%z = input(9,1);
phi = input(10,1);
theta = input(11,1);
Psi = input(12,1);

DOF6 = 1; % Select degrees of freedom

tmp1 = []; tmp2 = [];

if DOF6 == 1
    
    % Rotation matrix
    R_x_phi = [1 0 0; 0 cos(phi) sin(phi); 0 -sin(phi) cos(phi)];
    R_y_theta = [cos(theta) 0 -sin(theta); 0 1 0; sin(theta) 0 cos(theta)];% Provjeri matrice
    R_z_psi = [cos(Psi) sin(Psi) 0; -sin(Psi) cos(Psi) 0; 0 0 1];
    
    % Linear velocity transform
    J1 = R_z_psi.'*R_y_theta.'*R_x_phi.';
    
    % Angular velocity transform    
    tmp1 = R_x_phi(:,2);
    tmp1 = [0 0 0; tmp1.'; 0 0 0].';
    
    tmp2 = R_x_phi*R_y_theta;
    tmp2 = tmp2(:,3);
    tmp2 = [0 0 0; 0 0 0; tmp2.'].';
    
    J2 = inv(diag([1 0 0])+tmp1+tmp2);
    
elseif DOF6 == 0
    
    % Rotation matrix
    R_x_phi = eye(3);
    R_y_theta = eye(3);
    R_z_psi = [cos(Psi) sin(Psi) 0; -sin(Psi) cos(Psi) 0; 0 0 1]; % Provjeri matrice
    
    % Linear velocity transform
    J1 = R_z_psi.'*R_y_theta.'*R_x_phi.';
    
    % Angular velocity transform 
    tmp1 = R_x_phi(:,2);
    tmp1 = [0 0 0; tmp1.'; 0 0 0].';
    
    tmp2 = R_x_phi*R_y_theta;
    tmp2 = tmp2(:,3);
    tmp2 = [0 0 0; 0 0 0; tmp2.'].';
    
    J2 = inv(diag([1 0 0])+tmp1+tmp2);
    
end

eta1 = J1*[u v w].';
eta2 = J2*[p q r].';


y = [eta1.' eta2.'].';

== matlab function cmmi_lib/CMMI USV MODEL/Subsystem/wrap ==
  data: e input; ew output
function ew = wrap(e)

ew = mod(e, 2*pi);

if ew > pi
   ew = -2*pi + ew;
elseif ew <= -pi 
   ew = 2*pi + ew;
end

== matlab function cmmi_lib/Allocation2/MATLAB Function ==
  data: u input; y output
function y = fcn(u)

y = t200_inv(u);

== matlab function cmmi_lib/CMMI USV ROS/MATLAB Function2 ==
  data: is_new input; b output; rc_in input Bus: SL_Bus_std_msgs_Int8MultiArray
function b = fcn(is_new, rc_in)
    persistent buttons

    if isempty(buttons)
        buttons = [0 0 0 0 0 0 0 0]';
    end
    if is_new
        buttons(1) = double(rc_in.data(1)) < -0.2;
        buttons(2) = double(rc_in.data(2)) > 0.2;
    end
    b = buttons;
end
